simulink model "Vehicle_Resistance_Forces_Model"  (R2020a)
settings: Solver=VariableStepAuto  StartTime=0.0  StopTime=10.0  RelTol=1e-3
undefined symbols (not defined in the file): h, km, m, s
libraries: simulink x1, aerolibconvert2 x1
settings Model: Creator=akash  LastModifiedBy=akash

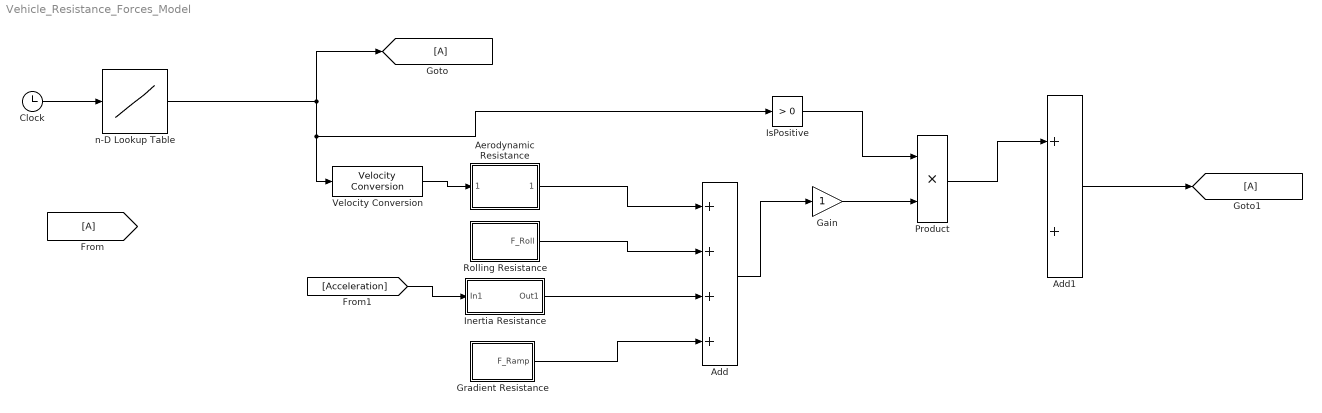
== system Vehicle_Resistance_Forces_Model ==
  Add : Sum  Inputs=++++
  Add1 : Sum
  Aerodynamic Resistance : Subsystem
  Clock : Clock
  Gain : Gain
  Gradient Resistance : Subsystem
  Inertia Resistance : Subsystem
  IsPositive : simulink/Logic and Bit Operations/Compare To Zero  relop=>  OutDataTypeStr=boolean
  Product : Product
  Rolling Resistance : Subsystem
  Velocity Conversion : aerolibconvert2/Velocity Conversion  IU=km/h  OU=m/s
  n-D Lookup Table : Lookup_n-D  NumberOfTableDimensions=1  DataSpecification=Lookup table object  LookupTableObject=sdf  BreakpointsForDimension3=[5, 7]  Table=4  InternalRulePriority=Speed  RndMeth=Simplest  InputSameDT=on
  wires:
  Clock/1 -> n-D Lookup Table/1
  Gain/1 -> Product/2
  Product/1 -> Add1/1
  Add/1 -> Gain/1
  Add1/1 -> [A]
  IsPositive/1 -> Product/1
  n-D Lookup Table/1 -> Velocity Conversion/1, IsPositive/1, [A]
  Velocity Conversion/1 -> Aerodynamic Resistance/1(Speed)
  Aerodynamic Resistance/1(F_Aero) -> Add/1
  Rolling Resistance/1(F_Roll) -> Add/2
  [Acceleration] -> Inertia Resistance/1(In1)
  Inertia Resistance/1(Out1) -> Add/3
  Gradient Resistance/1(F_Ramp) -> Add/4

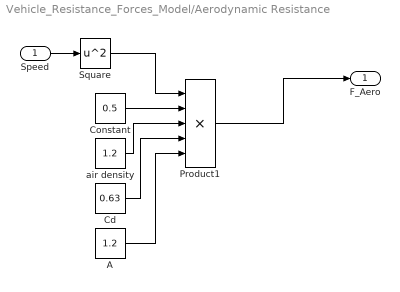
== system Vehicle_Resistance_Forces_Model/Aerodynamic Resistance ==
  Speed : Inport
  A : Constant  Value=1.2
  Cd : Constant  Value=0.63
  Constant : Constant  Value=0.5
  Product1 : Product  Inputs=5
  Square : Math  Operator=square  SaturateOnIntegerOverflow=on
  air density : Constant  Value=1.2
  F_Aero : Outport
  wires:
  air density/1 -> Product1/3
  Product1/1 -> F_Aero/1
  A/1 -> Product1/5
  Speed/1 -> Square/1
  Cd/1 -> Product1/4
  Constant/1 -> Product1/2
  Square/1 -> Product1/1

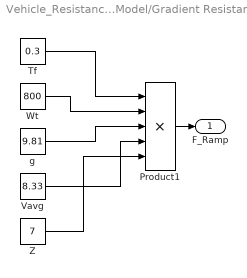
== system Vehicle_Resistance_Forces_Model/Gradient Resistance ==
  Product1 : Product  Inputs=5
  Tf : Constant  Value=0.3  VectorParams1D=off  SampleTime=-1
  Vavg : Constant  Value=8.33  VectorParams1D=off  SampleTime=-1
  Wt : Constant  Value=800  VectorParams1D=off  SampleTime=-1
  Z : Constant  Value=7  VectorParams1D=off  SampleTime=-1
  g : Constant  Value=9.81  VectorParams1D=off  SampleTime=-1
  F_Ramp : Outport
  wires:
  g/1 -> Product1/3
  Z/1 -> Product1/5
  Vavg/1 -> Product1/4
  Tf/1 -> Product1/1
  Product1/1 -> F_Ramp/1
  Wt/1 -> Product1/2

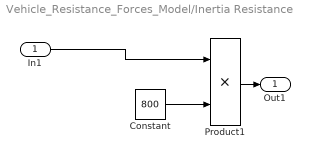
== system Vehicle_Resistance_Forces_Model/Inertia Resistance ==
  In1 : Inport
  Constant : Constant  Value=800
  Product1 : Product
  Out1 : Outport
  wires:
  Constant/1 -> Product1/2
  In1/1 -> Product1/1
  Product1/1 -> Out1/1

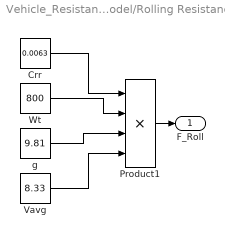
== system Vehicle_Resistance_Forces_Model/Rolling Resistance ==
  Crr : Constant  Value=0.0063
  Product1 : Product  Inputs=4
  Vavg : Constant  Value=8.33
  Wt : Constant  Value=800
  g : Constant  Value=9.81
  F_Roll : Outport
  wires:
  g/1 -> Product1/3
  Crr/1 -> Product1/1
  Vavg/1 -> Product1/4
  Wt/1 -> Product1/2
  Product1/1 -> F_Roll/1
